simulink model "bic_4"  (R2018b)
settings: Solver=FixedStepAuto  StartTime=0.0  StopTime=1  FixedStep=Ts  RelTol=1e-5  EnableMultiTasking=on
values from neighbouring files (symbols this model uses):
  a_cmd = a    [sim_veh_MPC.m]    (also in sim_veh_MPC_smooth.m)
  psi0 = psi    (= 0)    [sim_veh_MPC.m]    (also in sim_veh_MPC_smooth.m)
  v_car0 = v    (= 5)    [sim_veh_MPC.m]    (also in sim_veh_MPC_smooth.m)
  x_car0 = x_car    (= 0)    [sim_veh_MPC.m]    (also in sim_veh_MPC_smooth.m)
  y_car0 = y_car    (= 0)    [sim_veh_MPC.m]    (also in sim_veh_MPC_smooth.m)
undefined symbols (not defined in the file or in its folder): alpha_car0, s_cmd
settings Model: Creator=Jesse  LastModifiedBy=Bolin.zhao
settings DataIOCC: LimitDataPoints=on
settings OptimizationCC: LifeSpan=inf
settings DebuggingCC: AllowSymbolicDim=off  LibraryContextMissingDiagnostic=none  SFUnexpectedBacktrackingDiag=warning  SFNoUnconditionalDefaultTransitionDiag=warning  SFExecutionAtInitializationDiag=none
settings ModelReferenceCC: PropagateSignalLabelsOutOfModel=off
settings SFSimCC: SimUseLocalCustomCode=off
settings RTWCC: RTWUseLocalCustomCode=off
settings CodeAppCC: StateflowObjectComments=on
settings GRTTargetCC: TargetLangStandard=C89/C90 (ANSI)
settings ConfigComp: CovMetricSettings=dw  CovHtmlReporting=on  CovSaveCumulativeToWorkspaceVar=on  CovSaveSingleToWorkspaceVar=on  CovExternalEMLEnable=off

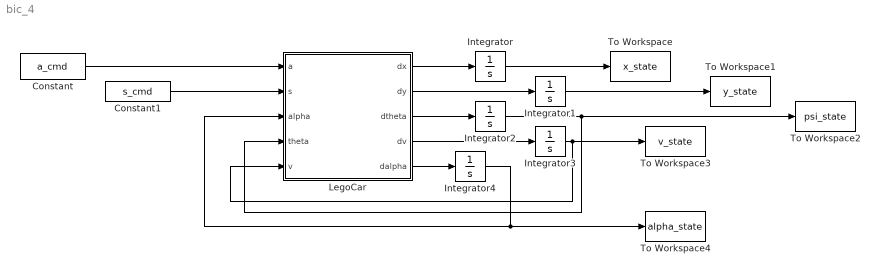
== system bic_4 ==
  Constant : Constant  Value=a_cmd
  Constant1 : Constant  Value=s_cmd
  Integrator : Integrator  InitialCondition=x_car0
  Integrator1 : Integrator  InitialCondition=y_car0
  Integrator2 : Integrator  InitialCondition=psi0
  Integrator3 : Integrator  InitialCondition=v_car0
  Integrator4 : Integrator  InitialCondition=alpha_car0
  LegoCar : MATLAB Function  TreatAsAtomicUnit=on
  To Workspace : ToWorkspace  VariableName=x_state  SaveFormat=Timeseries  SampleTime=-1
  To Workspace1 : ToWorkspace  VariableName=y_state  SaveFormat=Timeseries  SampleTime=-1
  To Workspace2 : ToWorkspace  VariableName=psi_state  SaveFormat=Timeseries  SampleTime=-1
  To Workspace3 : ToWorkspace  VariableName=v_state  SaveFormat=Timeseries  SampleTime=-1
  To Workspace4 : ToWorkspace  VariableName=alpha_state  SaveFormat=Timeseries  SampleTime=-1
  wires:
  LegoCar/3(dtheta) -> Integrator2/1
  Integrator2/1 -> LegoCar/4(theta), To Workspace2/1
  LegoCar/2(dy) -> Integrator1/1
  LegoCar/1(dx) -> Integrator/1
  Constant/1 -> LegoCar/1(a)
  Integrator/1 -> To Workspace/1
  Integrator1/1 -> To Workspace1/1
  LegoCar/4(dv) -> Integrator3/1
  Integrator3/1 -> LegoCar/5(v), To Workspace3/1
  Constant1/1 -> LegoCar/2(s)
  LegoCar/5(dalpha) -> Integrator4/1
  Integrator4/1 -> LegoCar/3(alpha), To Workspace4/1

== matlab function bic_4/LegoCar ==
  data: a input; s input; dx output; alpha input; theta input; dy output; dtheta output; dv output; v input; dalpha output
function [dx,dy,dtheta,dv,dalpha] = fcn(a,s,alpha,theta,v)
% this model add the steering angle state
%[aplha] current steering wheel angle
%[theta] heading angle

lr = 1.7;
lf = 1.5;
beta = atan(lr/(lr+lf)*tan(alpha));
dx = v*cos(theta+beta);
dy = v*sin(theta+beta);
dtheta = v/lr*tan(beta);
dv = a;
dalpha = s;
